simulink model "Lab1_Part3"  (R2022b)
settings: Solver=VariableStepAuto  StartTime=0.0  StopTime=10  RelTol=1e-3
settings Model: Creator=Sahaj Singh  LastModifiedBy=rosie

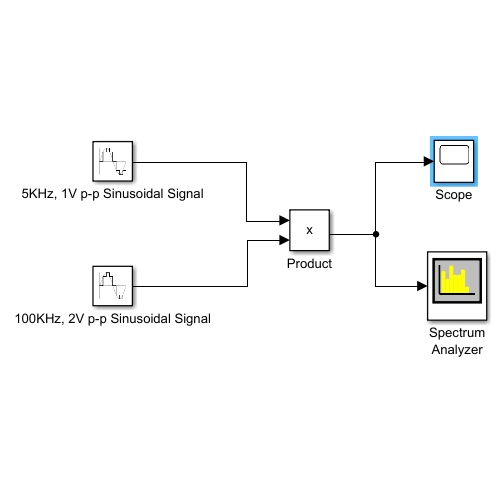
[thumbnail: Simulink's stored preview of the top-level diagram]
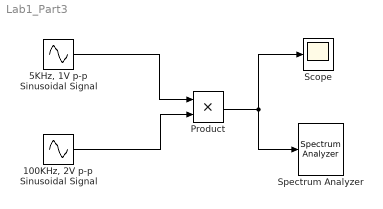
== system Lab1_Part3 ==
  "100KHz, 2V p-p Sinusoidal Signal" : Sin  Frequency=100000*2*pi  SampleTime=0.0000005
  "5KHz, 1V p-p Sinusoidal Signal" : Sin  Amplitude=0.5  Frequency=5000*2*pi  SampleTime=0.0000005
  Product : Product
  Scope : Scope
  Spectrum Analyzer : SpectrumAnalyzer
  wires:
  "5KHz, 1V p-p Sinusoidal Signal"/1 -> Product/1
  "100KHz, 2V p-p Sinusoidal Signal"/1 -> Product/2
  Product/1 -> Spectrum Analyzer/1, Scope/1
